simulink model "controller"  (R2023b)
settings: Solver=FixedStepAuto  StartTime=0.0  StopTime=10.0  FixedStep=1/100  RelTol=1e-3
undefined symbols (not defined in the file): MAX_TORQUE, MAX_TORQUE_REVERSE
settings Model: Creator=DAUIN-Win10  LastModifiedBy=Matteo
settings OptimizationCC: ReuseModelBlockBuffer=off
settings DebuggingCC: UnconnectedInputMsg=warning  UnconnectedOutputMsg=warning  UnconnectedLineMsg=warning
settings ModelReferenceCC: EnableRefExpFcnMdlSchedulingChecks=on
settings RTWCC: DLArmComputeVersion=19.05

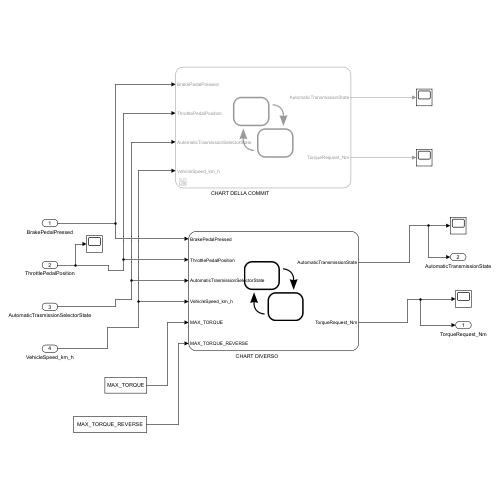
[thumbnail: Simulink's stored preview of the top-level diagram]
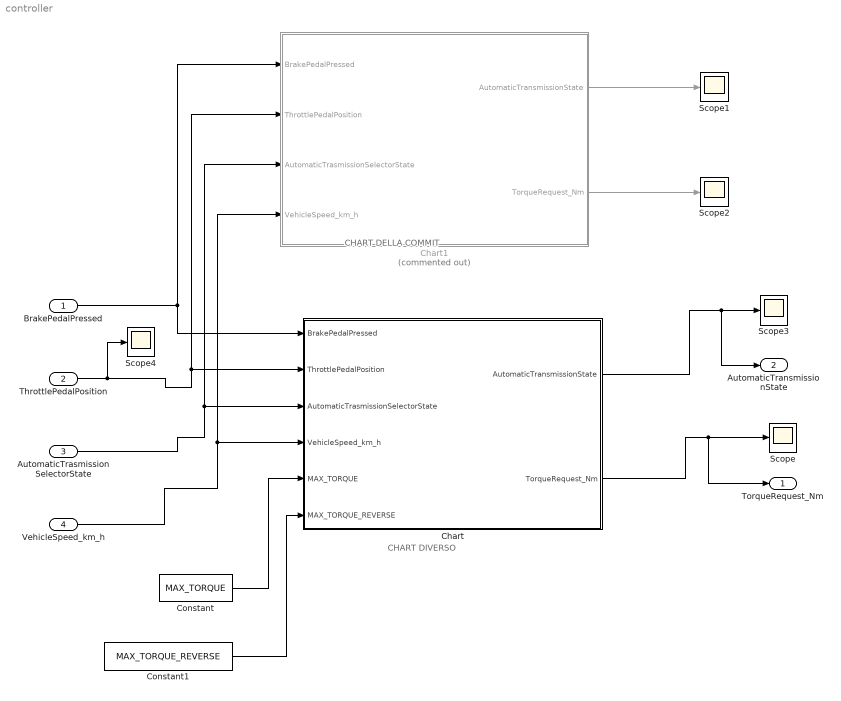
== system controller ==
  note: CHART DIVERSO
  note: CHART DELLA COMMIT
  BrakePedalPressed : Inport  OutDataTypeStr=boolean
  ThrottlePedalPosition : Inport  Port=2  OutDataTypeStr=single
  AutomaticTrasmissionSelectorState : Inport  Port=3  OutDataTypeStr=Enum: TransmissionState
  VehicleSpeed_km_h : Inport  Port=4  OutDataTypeStr=single  Unit=km/h
  Chart : Stateflow chart  TreatAsAtomicUnit=on
  Chart1 : Stateflow chart  Commented=on  TreatAsAtomicUnit=on
  Constant : Constant  Value=MAX_TORQUE
  Constant1 : Constant  Value=MAX_TORQUE_REVERSE
  Scope{,1..4} (5 alike) : Scope
  TorqueRequest_Nm : Outport  OutDataTypeStr=single  Unit=N*m
  AutomaticTransmissionState : Outport  Port=2  OutDataTypeStr=Enum: TransmissionState
  wires:
  BrakePedalPressed/1 -> Chart1/1(BrakePedalPressed), Chart/1(BrakePedalPressed)
  ThrottlePedalPosition/1 -> Scope4/1, Chart1/2(ThrottlePedalPosition), Chart/2(ThrottlePedalPosition)
  AutomaticTrasmissionSelectorState/1 -> Chart1/3(AutomaticTrasmissionSelectorState), Chart/3(AutomaticTrasmissionSelectorState)
  VehicleSpeed_km_h/1 -> Chart1/4(VehicleSpeed_km_h), Chart/4(VehicleSpeed_km_h)
  Chart/2(TorqueRequest_Nm) -> Scope/1, TorqueRequest_Nm/1
  Chart/1(AutomaticTransmissionState) -> Scope3/1, AutomaticTransmissionState/1
  Chart1/2(TorqueRequest_Nm) -> Scope2/1
  Chart1/1(AutomaticTransmissionState) -> Scope1/1
  Constant/1 -> Chart/5(MAX_TORQUE)
  Constant1/1 -> Chart/6(MAX_TORQUE_REVERSE)

== stateflow chart controller/Chart1 ==
  settings: executeAtInitialization=1
  state B
    AutomaticTransmissionState=TransmissionState.Brake;
    if(ThrottlePedalPosition > 1/3)
    TorqueRequest_Nm = 80 * (3/2) * (ThrottlePedalPosition-1/3);
    else
    TorqueRequest_Nm = -40 * (1-3*ThrottlePedalPosition);
    end
  state P
    AutomaticTransmissionState=TransmissionState.Park;
    TorqueRequest_Nm = 0;
  state D
    AutomaticTransmissionState=TransmissionState.Drive;
    TorqueRequest_Nm = MAX_TORQUE*ThrottlePedalPosition;
  state N
    AutomaticTransmissionState=TransmissionState.Neutral;
    TorqueRequest_Nm = 0;
  state R
    AutomaticTransmissionState=TransmissionState.Reverse;
    TorqueRequest_Nm = -40*ThrottlePedalPosition;
  D -> B [order 1] : [ThrottlePedalPosition>1/3 && AutomaticTrasmissionSelectorState==TransmissionState.Brake]
  B -> D : [AutomaticTrasmissionSelectorState==TransmissionState.Drive]
  (default) -> P
  N -> P [order 3] : [AutomaticTrasmissionSelectorState==TransmissionState.Park && abs(VehicleSpeed_km_h)<5 && BrakePedalPressed==1]
  P -> N : [BrakePedalPressed==1 && AutomaticTrasmissionSelectorState==TransmissionState.Neutral]
  D -> N [order 2] : [AutomaticTrasmissionSelectorState==TransmissionState.Neutral]
  N -> R [order 1] : [VehicleSpeed_km_h<5 && BrakePedalPressed==1 && AutomaticTrasmissionSelectorState==TransmissionState.Reverse]
  N -> D [order 2] : [VehicleSpeed_km_h>-5 && BrakePedalPressed==1 && AutomaticTrasmissionSelectorState==TransmissionState.Drive]
  R -> N : [AutomaticTrasmissionSelectorState==TransmissionState.Neutral]
  data: BrakePedalPressed input; ThrottlePedalPosition input; AutomaticTrasmissionSelectorState input; VehicleSpeed_km_h input; AutomaticTransmissionState output; TorqueRequest_Nm output; MAX_TORQUE constant double

== stateflow chart controller/Chart ==
  settings: executeAtInitialization=1
  state BRAKE
    entry:
    AutomaticTransmissionState=TransmissionState.Brake;
    during:
    if(ThrottlePedalPosition > 1/3)
    TorqueRequest_Nm = MAX_TORQUE * (3/2) * (ThrottlePedalPosition-1/3);
    else
    TorqueRequest_Nm = -MAX_TORQUE_REVERSE * (1-3*ThrottlePedalPosition);
    end
  state PARK
    entry:
    AutomaticTransmissionState=TransmissionState.Park;
    during:
    TorqueRequest_Nm = 0;
  state DRIVE
    entry:
    AutomaticTransmissionState=TransmissionState.Drive;
    during:
    TorqueRequest_Nm = MAX_TORQUE*ThrottlePedalPosition;
  state NEUTRAL
    entry:
    AutomaticTransmissionState=TransmissionState.Neutral;
    during:
    TorqueRequest_Nm = 0;
  state REVERSE
    entry:
    AutomaticTransmissionState=TransmissionState.Reverse;
    during:
    TorqueRequest_Nm = -MAX_TORQUE_REVERSE*ThrottlePedalPosition;
  DRIVE -> BRAKE [order 1] : [ThrottlePedalPosition>1/3 && AutomaticTrasmissionSelectorState>TransmissionState.Drive]
  BRAKE -> DRIVE : [AutomaticTrasmissionSelectorState<TransmissionState.Brake]
  (default) -> PARK
  NEUTRAL -> PARK [order 3] : [AutomaticTrasmissionSelectorState==TransmissionState.Park && abs(VehicleSpeed_km_h)<5 && BrakePedalPressed==1]
  PARK -> NEUTRAL : [BrakePedalPressed==1 && AutomaticTrasmissionSelectorState>TransmissionState.Park]
  DRIVE -> NEUTRAL [order 2] : [AutomaticTrasmissionSelectorState<TransmissionState.Drive]
  NEUTRAL -> REVERSE [order 1] : [VehicleSpeed_km_h<5 && BrakePedalPressed==1 && AutomaticTrasmissionSelectorState<TransmissionState.Neutral && AutomaticTrasmissionSelectorState>TransmissionState.Park]
  NEUTRAL -> DRIVE [order 2] : [VehicleSpeed_km_h>-5 && BrakePedalPressed==1 && AutomaticTrasmissionSelectorState>TransmissionState.Neutral]
  REVERSE -> NEUTRAL : [AutomaticTrasmissionSelectorState>TransmissionState.Reverse]
  data: BrakePedalPressed input; ThrottlePedalPosition input; AutomaticTrasmissionSelectorState input; VehicleSpeed_km_h input; AutomaticTransmissionState output; TorqueRequest_Nm output; MAX_TORQUE input; MAX_TORQUE_REVERSE input
